simulink model "fuzzy_controller_7_trimf"  (Simulink 7.2)
settings: Solver=ode45  StartTime=0.0  StopTime=10.0  RelTol=1e-3
values from neighbouring files (symbols this model uses):
  fi_1_a = -0.786    [fuzzy_controller_3_trimf_params.m]    (also in fuzzy_controller_5_gbell_params.m = 0.1768; fuzzy_controller_5_trimf_optimal_params.m; fuzzy_controller_5_trimf_params.m; fuzzy_controller_7_trimf_params.m)
  fi_1_b = -0.786    [fuzzy_controller_3_trimf_params.m]    (also in fuzzy_controller_5_gbell_params.m = 3.278; fuzzy_controller_5_trimf_optimal_params.m; fuzzy_controller_5_trimf_params.m; fuzzy_controller_7_trimf_params.m)
  fi_1_c = 0    [fuzzy_controller_3_trimf_params.m]    (also in fuzzy_controller_5_gbell_params.m = -0.7664; fuzzy_controller_5_trimf_optimal_params.m = -0.1; fuzzy_controller_5_trimf_params.m = -0.393; fuzzy_controller_7_trimf_params.m = -0.523)
  fi_2_a = -0.786    [fuzzy_controller_3_trimf_params.m]    (also in fuzzy_controller_5_gbell_params.m = 0.1965; fuzzy_controller_5_trimf_optimal_params.m = -0.1; fuzzy_controller_5_trimf_params.m; fuzzy_controller_7_trimf_params.m)
  fi_2_b = 0    [fuzzy_controller_3_trimf_params.m]    (also in fuzzy_controller_5_gbell_params.m = 3.278; fuzzy_controller_5_trimf_optimal_params.m = -0.05; fuzzy_controller_5_trimf_params.m = -0.393; fuzzy_controller_7_trimf_params.m = -0.5238)
  fi_2_c = 0.786    [fuzzy_controller_3_trimf_params.m]    (also in fuzzy_controller_5_gbell_params.m = -0.393; fuzzy_controller_5_trimf_optimal_params.m = 0; fuzzy_controller_5_trimf_params.m = 0; fuzzy_controller_7_trimf_params.m = -0.262)
  fi_3_a = 0    [fuzzy_controller_3_trimf_params.m]    (also in fuzzy_controller_5_gbell_params.m = 0.1965; fuzzy_controller_5_trimf_optimal_params.m = -0.05; fuzzy_controller_5_trimf_params.m = -0.393; fuzzy_controller_7_trimf_params.m = -0.523)
  fi_3_b = 0.786    [fuzzy_controller_3_trimf_params.m]    (also in fuzzy_controller_5_gbell_params.m = 3.278; fuzzy_controller_5_trimf_optimal_params.m = 0; fuzzy_controller_5_trimf_params.m = 0; fuzzy_controller_7_trimf_params.m = -0.262)
  fi_3_c = 0.786    [fuzzy_controller_3_trimf_params.m]    (also in fuzzy_controller_5_gbell_params.m = 0; fuzzy_controller_5_trimf_optimal_params.m = 0.05; fuzzy_controller_5_trimf_params.m = 0.393; fuzzy_controller_7_trimf_params.m = 0)
  fi_4_a = 0.1965    [fuzzy_controller_5_gbell_params.m]    (also in fuzzy_controller_5_trimf_optimal_params.m = 0; fuzzy_controller_5_trimf_params.m = 0; fuzzy_controller_7_trimf_params.m = -0.262)
  fi_4_b = 3.278    [fuzzy_controller_5_gbell_params.m]    (also in fuzzy_controller_5_trimf_optimal_params.m = 0.05; fuzzy_controller_5_trimf_params.m = 0.393; fuzzy_controller_7_trimf_params.m = 0)
  fi_4_c = 0.393    [fuzzy_controller_5_gbell_params.m]    (also in fuzzy_controller_5_trimf_optimal_params.m = 0.1; fuzzy_controller_5_trimf_params.m = 0.786; fuzzy_controller_7_trimf_params.m = 0.262)
  fi_5_a = 0.1768    [fuzzy_controller_5_gbell_params.m]    (also in fuzzy_controller_5_trimf_optimal_params.m = 0.05; fuzzy_controller_5_trimf_params.m = 0.393; fuzzy_controller_7_trimf_params.m = 0)
  fi_5_b = 3.278    [fuzzy_controller_5_gbell_params.m]    (also in fuzzy_controller_5_trimf_optimal_params.m = 0.1; fuzzy_controller_5_trimf_params.m = 0.786; fuzzy_controller_7_trimf_params.m = 0.262)
  fi_5_c = 0.7664    [fuzzy_controller_5_gbell_params.m]    (also in fuzzy_controller_5_trimf_optimal_params.m = 0.786; fuzzy_controller_5_trimf_params.m = 0.786; fuzzy_controller_7_trimf_params.m = 0.523)
  fi_6_a = 0.262    [fuzzy_controller_7_trimf_params.m]
  fi_6_b = 0.523    [fuzzy_controller_7_trimf_params.m]
  fi_6_c = 0.786    [fuzzy_controller_7_trimf_params.m]
  fi_7_a = 0.523    [fuzzy_controller_7_trimf_params.m]
  fi_7_b = 0.786    [fuzzy_controller_7_trimf_params.m]
  fi_7_c = 0.786    [fuzzy_controller_7_trimf_params.m]
  FORCE_1_a = -150    [fuzzy_controller_3_trimf_params.m]    (also in fuzzy_controller_5_trimf_optimal_params.m; fuzzy_controller_5_trimf_params.m; fuzzy_controller_7_trimf_params.m)
  FORCE_1_b = -150    [fuzzy_controller_3_trimf_params.m]    (also in fuzzy_controller_5_trimf_optimal_params.m; fuzzy_controller_5_trimf_params.m; fuzzy_controller_7_trimf_params.m)
  FORCE_1_c = 0    [fuzzy_controller_3_trimf_params.m]    (also in fuzzy_controller_5_trimf_optimal_params.m = -75; fuzzy_controller_5_trimf_params.m = -75; fuzzy_controller_7_trimf_params.m = -100)
  FORCE_2_a = -150    [fuzzy_controller_3_trimf_params.m]    (also in fuzzy_controller_5_trimf_optimal_params.m; fuzzy_controller_5_trimf_params.m; fuzzy_controller_7_trimf_params.m)
  FORCE_2_b = 0    [fuzzy_controller_3_trimf_params.m]    (also in fuzzy_controller_5_trimf_optimal_params.m = -75; fuzzy_controller_5_trimf_params.m = -75; fuzzy_controller_7_trimf_params.m = -100)
  FORCE_2_c = 150    [fuzzy_controller_3_trimf_params.m]    (also in fuzzy_controller_5_trimf_optimal_params.m = 0; fuzzy_controller_5_trimf_params.m = 0; fuzzy_controller_7_trimf_params.m = -50)
  FORCE_3_a = 0    [fuzzy_controller_3_trimf_params.m]    (also in fuzzy_controller_5_trimf_optimal_params.m = -75; fuzzy_controller_5_trimf_params.m = -75; fuzzy_controller_7_trimf_params.m = -100)
  FORCE_3_b = 150    [fuzzy_controller_3_trimf_params.m]    (also in fuzzy_controller_5_trimf_optimal_params.m = 0; fuzzy_controller_5_trimf_params.m = 0; fuzzy_controller_7_trimf_params.m = -50)
  FORCE_3_c = 150    [fuzzy_controller_3_trimf_params.m]    (also in fuzzy_controller_5_trimf_optimal_params.m = 75; fuzzy_controller_5_trimf_params.m = 75; fuzzy_controller_7_trimf_params.m = 0)
  FORCE_4_a = 0    [fuzzy_controller_5_trimf_optimal_params.m]    (also in fuzzy_controller_5_trimf_params.m; fuzzy_controller_7_trimf_params.m = -50)
  FORCE_4_b = 75    [fuzzy_controller_5_trimf_optimal_params.m]    (also in fuzzy_controller_5_trimf_params.m; fuzzy_controller_7_trimf_params.m = 0)
  FORCE_4_c = 150    [fuzzy_controller_5_trimf_optimal_params.m]    (also in fuzzy_controller_5_trimf_params.m; fuzzy_controller_7_trimf_params.m = 50)
  FORCE_5_a = 75    [fuzzy_controller_5_trimf_optimal_params.m]    (also in fuzzy_controller_5_trimf_params.m; fuzzy_controller_7_trimf_params.m = 0)
  FORCE_5_b = 150    [fuzzy_controller_5_trimf_optimal_params.m]    (also in fuzzy_controller_5_trimf_params.m; fuzzy_controller_7_trimf_params.m = 50)
  FORCE_5_c = 150    [fuzzy_controller_5_trimf_optimal_params.m]    (also in fuzzy_controller_5_trimf_params.m; fuzzy_controller_7_trimf_params.m = 100)
  FORCE_6_a = 50    [fuzzy_controller_7_trimf_params.m]
  FORCE_6_b = 100    [fuzzy_controller_7_trimf_params.m]
  FORCE_6_c = 150    [fuzzy_controller_7_trimf_params.m]
  FORCE_7_a = 100    [fuzzy_controller_7_trimf_params.m]
  FORCE_7_b = 150    [fuzzy_controller_7_trimf_params.m]
  FORCE_7_c = 150    [fuzzy_controller_7_trimf_params.m]
  FORCE_Range_1 = -150    [fuzzy_controller_3_trimf_params.m]    (also in fuzzy_controller_5_gauss_params.m; fuzzy_controller_5_gbell_params.m; fuzzy_controller_5_trimf_optimal_params.m; fuzzy_controller_5_trimf_params.m)
  FORCE_Range_2 = 150    [fuzzy_controller_3_trimf_params.m]    (also in fuzzy_controller_5_gauss_params.m; fuzzy_controller_5_gbell_params.m; fuzzy_controller_5_trimf_optimal_params.m; fuzzy_controller_5_trimf_params.m)
  omega_1_a = -1.57    [fuzzy_controller_3_trimf_params.m]    (also in fuzzy_controller_5_gbell_params.m = 0.3532; fuzzy_controller_5_trimf_optimal_params.m; fuzzy_controller_5_trimf_params.m; fuzzy_controller_7_trimf_params.m)
  omega_1_b = -1.57    [fuzzy_controller_3_trimf_params.m]    (also in fuzzy_controller_5_gbell_params.m = 3.278; fuzzy_controller_5_trimf_optimal_params.m; fuzzy_controller_5_trimf_params.m; fuzzy_controller_7_trimf_params.m)
  omega_1_c = 0    [fuzzy_controller_3_trimf_params.m]    (also in fuzzy_controller_5_gbell_params.m = -1.531; fuzzy_controller_5_trimf_optimal_params.m = -0.86; fuzzy_controller_5_trimf_params.m = -0.785; fuzzy_controller_7_trimf_params.m = -1.047)
  omega_2_a = -1.57    [fuzzy_controller_3_trimf_params.m]    (also in fuzzy_controller_5_gbell_params.m = 0.3925; fuzzy_controller_5_trimf_optimal_params.m = -0.86; fuzzy_controller_5_trimf_params.m; fuzzy_controller_7_trimf_params.m)
  omega_2_b = 0    [fuzzy_controller_3_trimf_params.m]    (also in fuzzy_controller_5_gbell_params.m = 3.278; fuzzy_controller_5_trimf_optimal_params.m = -0.43; fuzzy_controller_5_trimf_params.m = -0.785; fuzzy_controller_7_trimf_params.m = -1.047)
  omega_2_c = 1.57    [fuzzy_controller_3_trimf_params.m]    (also in fuzzy_controller_5_gbell_params.m = -0.785; fuzzy_controller_5_trimf_optimal_params.m = 0; fuzzy_controller_5_trimf_params.m = 0; fuzzy_controller_7_trimf_params.m = -0.523)
  omega_3_a = 0    [fuzzy_controller_3_trimf_params.m]    (also in fuzzy_controller_5_gbell_params.m = 0.3925; fuzzy_controller_5_trimf_optimal_params.m = -0.43; fuzzy_controller_5_trimf_params.m = -0.785; fuzzy_controller_7_trimf_params.m = -1.047)
  omega_3_b = 1.57    [fuzzy_controller_3_trimf_params.m]    (also in fuzzy_controller_5_gbell_params.m = 3.278; fuzzy_controller_5_trimf_optimal_params.m = 0; fuzzy_controller_5_trimf_params.m = 0; fuzzy_controller_7_trimf_params.m = -0.523)
  omega_3_c = 1.57    [fuzzy_controller_3_trimf_params.m]    (also in fuzzy_controller_5_gbell_params.m = 0; fuzzy_controller_5_trimf_optimal_params.m = 0.43; fuzzy_controller_5_trimf_params.m = 0.785; fuzzy_controller_7_trimf_params.m = 0)
  omega_4_a = 0.3925    [fuzzy_controller_5_gbell_params.m]    (also in fuzzy_controller_5_trimf_optimal_params.m = 0; fuzzy_controller_5_trimf_params.m = 0; fuzzy_controller_7_trimf_params.m = -0.523)
  omega_4_b = 3.278    [fuzzy_controller_5_gbell_params.m]    (also in fuzzy_controller_5_trimf_optimal_params.m = 0.43; fuzzy_controller_5_trimf_params.m = 0.785; fuzzy_controller_7_trimf_params.m = 0)
  omega_4_c = 0.785    [fuzzy_controller_5_gbell_params.m]    (also in fuzzy_controller_5_trimf_optimal_params.m = 0.86; fuzzy_controller_5_trimf_params.m = 1.57; fuzzy_controller_7_trimf_params.m = 0.523)
  omega_5_a = 0.3532    [fuzzy_controller_5_gbell_params.m]    (also in fuzzy_controller_5_trimf_optimal_params.m = 0.43; fuzzy_controller_5_trimf_params.m = 0.785; fuzzy_controller_7_trimf_params.m = 0)
  omega_5_b = 3.278    [fuzzy_controller_5_gbell_params.m]    (also in fuzzy_controller_5_trimf_optimal_params.m = 0.86; fuzzy_controller_5_trimf_params.m = 1.57; fuzzy_controller_7_trimf_params.m = 0.523)
  omega_5_c = 1.531    [fuzzy_controller_5_gbell_params.m]    (also in fuzzy_controller_5_trimf_optimal_params.m = 1.57; fuzzy_controller_5_trimf_params.m = 1.57; fuzzy_controller_7_trimf_params.m = 1.047)
  omega_6_a = 0.523    [fuzzy_controller_7_trimf_params.m]
  omega_6_b = 1.047    [fuzzy_controller_7_trimf_params.m]
  omega_6_c = 1.57    [fuzzy_controller_7_trimf_params.m]
  omega_7_a = 1.047    [fuzzy_controller_7_trimf_params.m]
  omega_7_b = 1.57    [fuzzy_controller_7_trimf_params.m]
  omega_7_c = 1.57    [fuzzy_controller_7_trimf_params.m]
(part 4 of 4)

== system fuzzy_controller_7_trimf/Fuzzy Logic Controller/omega/tri mf5 ==
  x : Inport
  0 : Constant  Value=0
  1 : Constant
  Constant : Constant  Value=a
  Constant1 : Constant  Value=c
  Constant2 : Constant  Value=b
  Constant3 : Constant  Value=0
  Logical Operator : Logic  Operator=OR  AllPortsSameDT=off  OutDataTypeMode=boolean  OutDataTypeStr=boolean
  Logical Operator1 : Logic  AllPortsSameDT=off  OutDataTypeMode=boolean  OutDataTypeStr=boolean
  Product ab (trimf) : Product  Inputs=*/  SaturateOnIntegerOverflow=on  InputSameDT=on  OutDataTypeStr=Inherit: Same as first input
  Product cd (trimf) : Product  Inputs=/*  SaturateOnIntegerOverflow=on  InputSameDT=on  OutDataTypeStr=Inherit: Same as first input
  Relational Operator : RelationalOperator  Operator=<  LogicOutDataTypeMode=boolean  OutDataTypeStr=boolean
  Relational Operator1 : RelationalOperator  Operator=>  LogicOutDataTypeMode=boolean  OutDataTypeStr=boolean
  Relational Operator2 : RelationalOperator  Operator===  LogicOutDataTypeMode=boolean  OutDataTypeStr=boolean
  Relational Operator3 : RelationalOperator  Operator=<  LogicOutDataTypeMode=boolean  OutDataTypeStr=boolean
  Relational Operator4 : RelationalOperator  Operator=>  LogicOutDataTypeMode=boolean  OutDataTypeStr=boolean
  Relational Operator5 : RelationalOperator  Operator=<=  LogicOutDataTypeMode=boolean  OutDataTypeStr=boolean
  Sum : Sum  Inputs=|+-  SaturateOnIntegerOverflow=on  InputSameDT=on  OutDataTypeStr=Inherit: Same as first input
  Sum1 : Sum  Inputs=-+  SaturateOnIntegerOverflow=on  InputSameDT=on  OutDataTypeStr=Inherit: Same as first input
  Sum2 : Sum  Inputs=-+  SaturateOnIntegerOverflow=on  InputSameDT=on  OutDataTypeStr=Inherit: Same as first input
  Sum3 : Sum  Inputs=+-  SaturateOnIntegerOverflow=on  InputSameDT=on  OutDataTypeStr=Inherit: Same as first input
  Sum4 : Sum  Inputs=++++
  Switch{,1..3} (4 alike) : Switch  Criteria=u2 > Threshold
  a : Constant  Value=a
  b : Constant  Value=b
  b1 : Constant  Value=b
  c : Constant  Value=c
  MF : Outport
  wires:
  0/1 -> Switch/1
  1/1 -> Switch1/1
  Constant/1 -> Relational Operator/2
  Relational Operator/1 -> Logical Operator/1
  Constant1/1 -> Relational Operator5/2, Relational Operator1/2
  Relational Operator1/1 -> Logical Operator/2
  Product ab (trimf)/1 -> Switch2/1  "(x-a)/(b-a)"
  a/1 -> Sum/2, Sum1/1
  b/1 -> Sum1/2
  Sum/1 -> Product ab (trimf)/1  "x-a"
  Sum1/1 -> Product ab (trimf)/2  "b-a"
  b1/1 -> Sum2/1
  x/1 -> Sum/1, Sum3/2, Relational Operator5/1, Relational Operator4/1, Relational Operator3/1, Relational Operator2/1, Relational Operator1/1, Relational Operator/1
  c/1 -> Sum3/1, Sum2/2
  Sum3/1 -> Product cd (trimf)/2  "c-x"
  Sum2/1 -> Product cd (trimf)/1  "c-b"
  Product cd (trimf)/1 -> Switch3/1  "(c-x)/(c-b)"
  Constant2/1 -> Relational Operator2/2, Relational Operator3/2, Relational Operator4/2
  Relational Operator4/1 -> Logical Operator1/1
  Relational Operator5/1 -> Logical Operator1/2
  Switch/1 -> Sum4/1
  Switch1/1 -> Sum4/2
  Switch2/1 -> Sum4/3
  Switch3/1 -> Sum4/4
  Constant3/1 -> Switch3/3, Switch2/3, Switch1/3, Switch/3
  Logical Operator1/1 -> Switch3/2
  Relational Operator3/1 -> Switch2/2
  Relational Operator2/1 -> Switch1/2
  Logical Operator/1 -> Switch/2
  Sum4/1 -> MF/1

== system fuzzy_controller_7_trimf/Fuzzy Logic Controller/omega/tri mf6 ==
  x : Inport
  0 : Constant  Value=0
  1 : Constant
  Constant : Constant  Value=a
  Constant1 : Constant  Value=c
  Constant2 : Constant  Value=b
  Constant3 : Constant  Value=0
  Logical Operator : Logic  Operator=OR  AllPortsSameDT=off  OutDataTypeMode=boolean  OutDataTypeStr=boolean
  Logical Operator1 : Logic  AllPortsSameDT=off  OutDataTypeMode=boolean  OutDataTypeStr=boolean
  Product ab (trimf) : Product  Inputs=*/  SaturateOnIntegerOverflow=on  InputSameDT=on  OutDataTypeStr=Inherit: Same as first input
  Product cd (trimf) : Product  Inputs=/*  SaturateOnIntegerOverflow=on  InputSameDT=on  OutDataTypeStr=Inherit: Same as first input
  Relational Operator : RelationalOperator  Operator=<  LogicOutDataTypeMode=boolean  OutDataTypeStr=boolean
  Relational Operator1 : RelationalOperator  Operator=>  LogicOutDataTypeMode=boolean  OutDataTypeStr=boolean
  Relational Operator2 : RelationalOperator  Operator===  LogicOutDataTypeMode=boolean  OutDataTypeStr=boolean
  Relational Operator3 : RelationalOperator  Operator=<  LogicOutDataTypeMode=boolean  OutDataTypeStr=boolean
  Relational Operator4 : RelationalOperator  Operator=>  LogicOutDataTypeMode=boolean  OutDataTypeStr=boolean
  Relational Operator5 : RelationalOperator  Operator=<=  LogicOutDataTypeMode=boolean  OutDataTypeStr=boolean
  Sum : Sum  Inputs=|+-  SaturateOnIntegerOverflow=on  InputSameDT=on  OutDataTypeStr=Inherit: Same as first input
  Sum1 : Sum  Inputs=-+  SaturateOnIntegerOverflow=on  InputSameDT=on  OutDataTypeStr=Inherit: Same as first input
  Sum2 : Sum  Inputs=-+  SaturateOnIntegerOverflow=on  InputSameDT=on  OutDataTypeStr=Inherit: Same as first input
  Sum3 : Sum  Inputs=+-  SaturateOnIntegerOverflow=on  InputSameDT=on  OutDataTypeStr=Inherit: Same as first input
  Sum4 : Sum  Inputs=++++
  Switch{,1..3} (4 alike) : Switch  Criteria=u2 > Threshold
  a : Constant  Value=a
  b : Constant  Value=b
  b1 : Constant  Value=b
  c : Constant  Value=c
  MF : Outport
  wires:
  0/1 -> Switch/1
  1/1 -> Switch1/1
  Constant/1 -> Relational Operator/2
  Relational Operator/1 -> Logical Operator/1
  Constant1/1 -> Relational Operator5/2, Relational Operator1/2
  Relational Operator1/1 -> Logical Operator/2
  Product ab (trimf)/1 -> Switch2/1  "(x-a)/(b-a)"
  a/1 -> Sum/2, Sum1/1
  b/1 -> Sum1/2
  Sum/1 -> Product ab (trimf)/1  "x-a"
  Sum1/1 -> Product ab (trimf)/2  "b-a"
  b1/1 -> Sum2/1
  x/1 -> Sum/1, Sum3/2, Relational Operator5/1, Relational Operator4/1, Relational Operator3/1, Relational Operator2/1, Relational Operator1/1, Relational Operator/1
  c/1 -> Sum3/1, Sum2/2
  Sum3/1 -> Product cd (trimf)/2  "c-x"
  Sum2/1 -> Product cd (trimf)/1  "c-b"
  Product cd (trimf)/1 -> Switch3/1  "(c-x)/(c-b)"
  Constant2/1 -> Relational Operator2/2, Relational Operator3/2, Relational Operator4/2
  Relational Operator4/1 -> Logical Operator1/1
  Relational Operator5/1 -> Logical Operator1/2
  Switch/1 -> Sum4/1
  Switch1/1 -> Sum4/2
  Switch2/1 -> Sum4/3
  Switch3/1 -> Sum4/4
  Constant3/1 -> Switch3/3, Switch2/3, Switch1/3, Switch/3
  Logical Operator1/1 -> Switch3/2
  Relational Operator3/1 -> Switch2/2
  Relational Operator2/1 -> Switch1/2
  Logical Operator/1 -> Switch/2
  Sum4/1 -> MF/1

== system fuzzy_controller_7_trimf/Fuzzy Logic Controller/omega/tri mf7 ==
  x : Inport
  0 : Constant  Value=0
  1 : Constant
  Constant : Constant  Value=a
  Constant1 : Constant  Value=c
  Constant2 : Constant  Value=b
  Constant3 : Constant  Value=0
  Logical Operator : Logic  Operator=OR  AllPortsSameDT=off  OutDataTypeMode=boolean  OutDataTypeStr=boolean
  Logical Operator1 : Logic  AllPortsSameDT=off  OutDataTypeMode=boolean  OutDataTypeStr=boolean
  Product ab (trimf) : Product  Inputs=*/  SaturateOnIntegerOverflow=on  InputSameDT=on  OutDataTypeStr=Inherit: Same as first input
  Product cd (trimf) : Product  Inputs=/*  SaturateOnIntegerOverflow=on  InputSameDT=on  OutDataTypeStr=Inherit: Same as first input
  Relational Operator : RelationalOperator  Operator=<  LogicOutDataTypeMode=boolean  OutDataTypeStr=boolean
  Relational Operator1 : RelationalOperator  Operator=>  LogicOutDataTypeMode=boolean  OutDataTypeStr=boolean
  Relational Operator2 : RelationalOperator  Operator===  LogicOutDataTypeMode=boolean  OutDataTypeStr=boolean
  Relational Operator3 : RelationalOperator  Operator=<  LogicOutDataTypeMode=boolean  OutDataTypeStr=boolean
  Relational Operator4 : RelationalOperator  Operator=>  LogicOutDataTypeMode=boolean  OutDataTypeStr=boolean
  Relational Operator5 : RelationalOperator  Operator=<=  LogicOutDataTypeMode=boolean  OutDataTypeStr=boolean
  Sum : Sum  Inputs=|+-  SaturateOnIntegerOverflow=on  InputSameDT=on  OutDataTypeStr=Inherit: Same as first input
  Sum1 : Sum  Inputs=-+  SaturateOnIntegerOverflow=on  InputSameDT=on  OutDataTypeStr=Inherit: Same as first input
  Sum2 : Sum  Inputs=-+  SaturateOnIntegerOverflow=on  InputSameDT=on  OutDataTypeStr=Inherit: Same as first input
  Sum3 : Sum  Inputs=+-  SaturateOnIntegerOverflow=on  InputSameDT=on  OutDataTypeStr=Inherit: Same as first input
  Sum4 : Sum  Inputs=++++
  Switch{,1..3} (4 alike) : Switch  Criteria=u2 > Threshold
  a : Constant  Value=a
  b : Constant  Value=b
  b1 : Constant  Value=b
  c : Constant  Value=c
  MF : Outport
  wires:
  0/1 -> Switch/1
  1/1 -> Switch1/1
  Constant/1 -> Relational Operator/2
  Relational Operator/1 -> Logical Operator/1
  Constant1/1 -> Relational Operator5/2, Relational Operator1/2
  Relational Operator1/1 -> Logical Operator/2
  Product ab (trimf)/1 -> Switch2/1  "(x-a)/(b-a)"
  a/1 -> Sum/2, Sum1/1
  b/1 -> Sum1/2
  Sum/1 -> Product ab (trimf)/1  "x-a"
  Sum1/1 -> Product ab (trimf)/2  "b-a"
  b1/1 -> Sum2/1
  x/1 -> Sum/1, Sum3/2, Relational Operator5/1, Relational Operator4/1, Relational Operator3/1, Relational Operator2/1, Relational Operator1/1, Relational Operator/1
  c/1 -> Sum3/1, Sum2/2
  Sum3/1 -> Product cd (trimf)/2  "c-x"
  Sum2/1 -> Product cd (trimf)/1  "c-b"
  Product cd (trimf)/1 -> Switch3/1  "(c-x)/(c-b)"
  Constant2/1 -> Relational Operator2/2, Relational Operator3/2, Relational Operator4/2
  Relational Operator4/1 -> Logical Operator1/1
  Relational Operator5/1 -> Logical Operator1/2
  Switch/1 -> Sum4/1
  Switch1/1 -> Sum4/2
  Switch2/1 -> Sum4/3
  Switch3/1 -> Sum4/4
  Constant3/1 -> Switch3/3, Switch2/3, Switch1/3, Switch/3
  Logical Operator1/1 -> Switch3/2
  Relational Operator3/1 -> Switch2/2
  Relational Operator2/1 -> Switch1/2
  Logical Operator/1 -> Switch/2
  Sum4/1 -> MF/1
